simulink model "fault_tolerant_controller_2014"  (R2014a)
settings: Solver=ode45  SolverMode=SingleTasking  StartTime=0.0  StopTime=150  RelTol=1e-3
values from neighbouring files (symbols this model uses):
  g = 9.8    [model.mat]
  Kd = 1e-06    [model.mat]
  Kt = 1    [model.mat]
  U0 = 120    [model.mat]
  X0 = 0    [model.mat]
  Y0 = 5000    [model.mat]
undefined symbols (not defined in the file or in its folder): magnitude
libraries: simulink x53, aerolibatmos2 x12, aerolibconvert2 x4
(part 2 of 2)

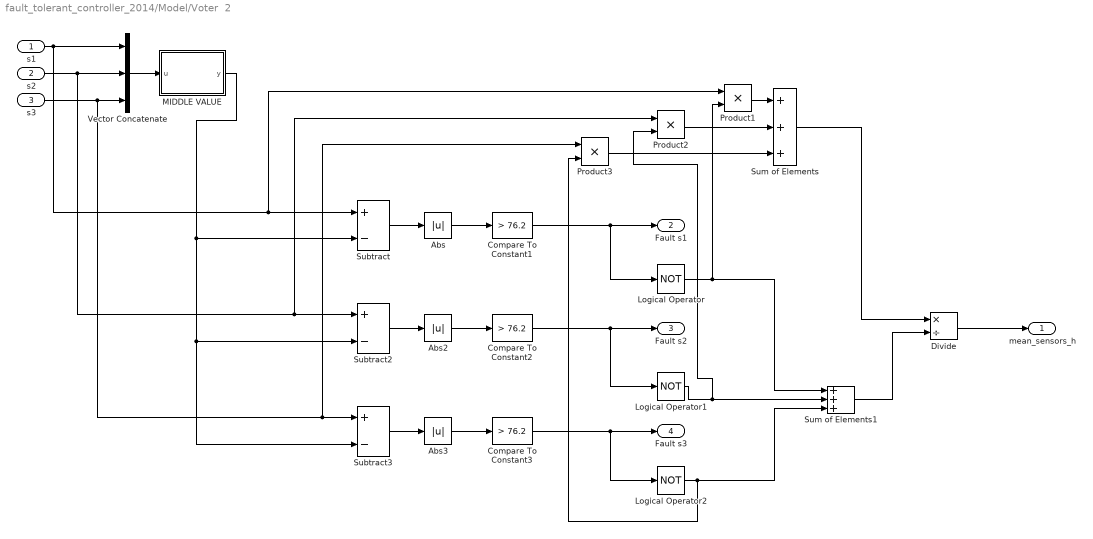
== system fault_tolerant_controller_2014/Model/Voter  2 ==
  s1 : Inport
  s2 : Inport  Port=2
  s3 : Inport  Port=3
  Abs : Abs
  Abs2 : Abs
  Abs3 : Abs
  Compare To Constant1 : simulink/Logic and Bit Operations/Compare To Constant  relop=>  const=76.2  OutDataTypeStr=boolean
  Compare To Constant2 : simulink/Logic and Bit Operations/Compare To Constant  relop=>  const=76.2  OutDataTypeStr=boolean
  Compare To Constant3 : simulink/Logic and Bit Operations/Compare To Constant  relop=>  const=76.2  OutDataTypeStr=boolean
  Divide : Product  Inputs=*/
  Logical Operator : Logic  Operator=NOT  AllPortsSameDT=off  OutDataTypeStr=boolean
  Logical Operator1 : Logic  Operator=NOT  AllPortsSameDT=off  OutDataTypeStr=boolean
  Logical Operator2 : Logic  Operator=NOT  AllPortsSameDT=off  OutDataTypeStr=boolean
  "MIDDLE VALUE " : MATLAB Function  TreatAsAtomicUnit=on
      settings: PermitHierarchicalResolution=ParametersOnly
  Product1 : Product
  Product2 : Product
  Product3 : Product
  Subtract : Sum  Inputs=+-
  Subtract2 : Sum  Inputs=+-
  Subtract3 : Sum  Inputs=+-
  Sum of Elements : Sum  Inputs=+++
  Sum of Elements1 : Sum  Inputs=+++
  Vector Concatenate : Concatenate  NumInputs=3
  " mean_sensors_h" : Outport
  "Fault s1  " : Outport  Port=2
  "Fault s2  " : Outport  Port=3
  "Fault s3  " : Outport  Port=4
  wires:
  Vector Concatenate/1 -> "MIDDLE VALUE "/1(u)
  Subtract3/1 -> Abs3/1
  Subtract/1 -> Abs/1
  s3/1 -> Product3/1, Subtract3/1, Vector Concatenate/3
  Subtract2/1 -> Abs2/1
  "MIDDLE VALUE "/1(y) -> Subtract/2, Subtract3/2, Subtract2/2
  Sum of Elements/1 -> Divide/1
  Sum of Elements1/1 -> Divide/2
  Divide/1 -> " mean_sensors_h"/1
  Abs/1 -> Compare To Constant1/1
  Compare To Constant1/1 -> Logical Operator/1, "Fault s1  "/1
  Compare To Constant2/1 -> Logical Operator1/1, "Fault s2  "/1
  Abs2/1 -> Compare To Constant2/1
  Abs3/1 -> Compare To Constant3/1
  Compare To Constant3/1 -> Logical Operator2/1, "Fault s3  "/1
  Logical Operator/1 -> Product1/2, Sum of Elements1/1
  Logical Operator1/1 -> Sum of Elements1/2, Product2/2
  Logical Operator2/1 -> Sum of Elements1/3, Product3/2
  s1/1 -> Product1/1, Subtract/1, Vector Concatenate/1
  s2/1 -> Product2/1, Subtract2/1, Vector Concatenate/2
  Product2/1 -> Sum of Elements/2
  Product3/1 -> Sum of Elements/3
  Product1/1 -> Sum of Elements/1

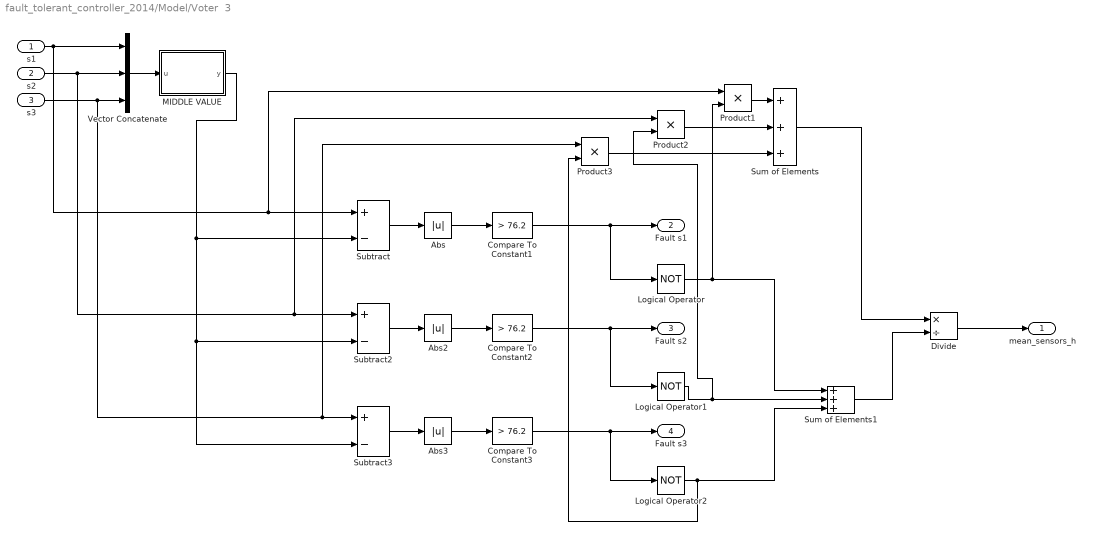
== system fault_tolerant_controller_2014/Model/Voter  3 ==
  s1 : Inport
  s2 : Inport  Port=2
  s3 : Inport  Port=3
  Abs : Abs
  Abs2 : Abs
  Abs3 : Abs
  Compare To Constant1 : simulink/Logic and Bit Operations/Compare To Constant  relop=>  const=76.2  OutDataTypeStr=boolean
  Compare To Constant2 : simulink/Logic and Bit Operations/Compare To Constant  relop=>  const=76.2  OutDataTypeStr=boolean
  Compare To Constant3 : simulink/Logic and Bit Operations/Compare To Constant  relop=>  const=76.2  OutDataTypeStr=boolean
  Divide : Product  Inputs=*/
  Logical Operator : Logic  Operator=NOT  AllPortsSameDT=off  OutDataTypeStr=boolean
  Logical Operator1 : Logic  Operator=NOT  AllPortsSameDT=off  OutDataTypeStr=boolean
  Logical Operator2 : Logic  Operator=NOT  AllPortsSameDT=off  OutDataTypeStr=boolean
  "MIDDLE VALUE " : MATLAB Function  TreatAsAtomicUnit=on
      settings: PermitHierarchicalResolution=ParametersOnly
  Product1 : Product
  Product2 : Product
  Product3 : Product
  Subtract : Sum  Inputs=+-
  Subtract2 : Sum  Inputs=+-
  Subtract3 : Sum  Inputs=+-
  Sum of Elements : Sum  Inputs=+++
  Sum of Elements1 : Sum  Inputs=+++
  Vector Concatenate : Concatenate  NumInputs=3
  " mean_sensors_h" : Outport
  "Fault s1  " : Outport  Port=2
  "Fault s2  " : Outport  Port=3
  "Fault s3  " : Outport  Port=4
  wires:
  Vector Concatenate/1 -> "MIDDLE VALUE "/1(u)
  Subtract3/1 -> Abs3/1
  Subtract/1 -> Abs/1
  s3/1 -> Product3/1, Subtract3/1, Vector Concatenate/3
  Subtract2/1 -> Abs2/1
  "MIDDLE VALUE "/1(y) -> Subtract/2, Subtract3/2, Subtract2/2
  Sum of Elements/1 -> Divide/1
  Sum of Elements1/1 -> Divide/2
  Divide/1 -> " mean_sensors_h"/1
  Abs/1 -> Compare To Constant1/1
  Compare To Constant1/1 -> Logical Operator/1, "Fault s1  "/1
  Compare To Constant2/1 -> Logical Operator1/1, "Fault s2  "/1
  Abs2/1 -> Compare To Constant2/1
  Abs3/1 -> Compare To Constant3/1
  Compare To Constant3/1 -> Logical Operator2/1, "Fault s3  "/1
  Logical Operator/1 -> Product1/2, Sum of Elements1/1
  Logical Operator1/1 -> Sum of Elements1/2, Product2/2
  Logical Operator2/1 -> Sum of Elements1/3, Product3/2
  s1/1 -> Product1/1, Subtract/1, Vector Concatenate/1
  s2/1 -> Product2/1, Subtract2/1, Vector Concatenate/2
  Product2/1 -> Sum of Elements/2
  Product3/1 -> Sum of Elements/3
  Product1/1 -> Sum of Elements/1

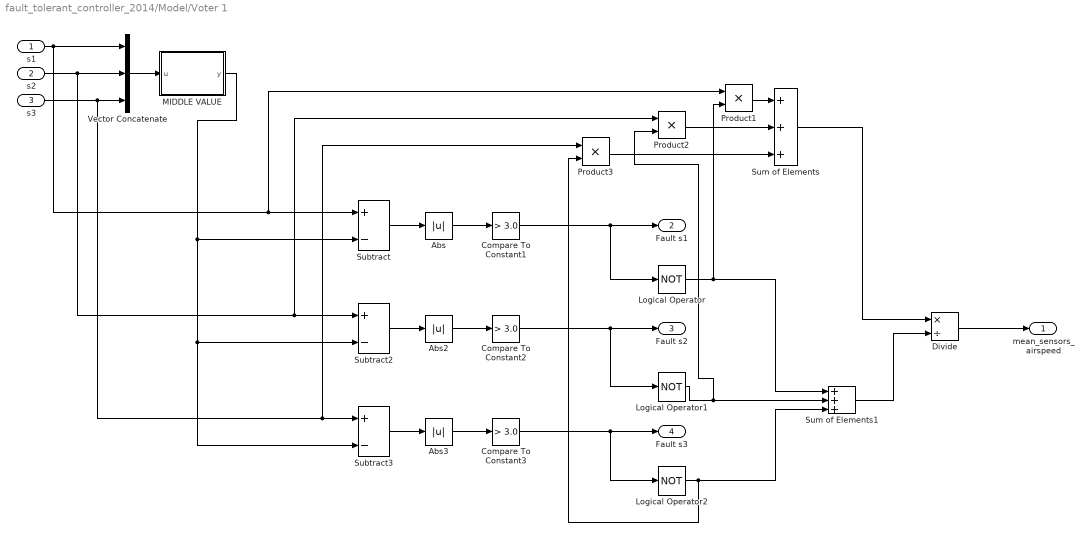
== system fault_tolerant_controller_2014/Model/Voter 1 ==
  s1 : Inport
  s2 : Inport  Port=2
  s3 : Inport  Port=3
  Abs : Abs
  Abs2 : Abs
  Abs3 : Abs
  Compare To Constant1 : simulink/Logic and Bit Operations/Compare To Constant  relop=>  const=3.0  OutDataTypeStr=boolean
  Compare To Constant2 : simulink/Logic and Bit Operations/Compare To Constant  relop=>  const=3.0  OutDataTypeStr=boolean
  Compare To Constant3 : simulink/Logic and Bit Operations/Compare To Constant  relop=>  const=3.0  OutDataTypeStr=boolean
  Divide : Product  Inputs=*/
  Logical Operator : Logic  Operator=NOT  AllPortsSameDT=off  OutDataTypeStr=boolean
  Logical Operator1 : Logic  Operator=NOT  AllPortsSameDT=off  OutDataTypeStr=boolean
  Logical Operator2 : Logic  Operator=NOT  AllPortsSameDT=off  OutDataTypeStr=boolean
  "MIDDLE VALUE " : MATLAB Function  TreatAsAtomicUnit=on
      settings: PermitHierarchicalResolution=ParametersOnly
  Product1 : Product
  Product2 : Product
  Product3 : Product
  Subtract : Sum  Inputs=+-
  Subtract2 : Sum  Inputs=+-
  Subtract3 : Sum  Inputs=+-
  Sum of Elements : Sum  Inputs=+++
  Sum of Elements1 : Sum  Inputs=+++
  Vector Concatenate : Concatenate  NumInputs=3
  " mean_sensors_airspeed" : Outport
  "Fault s1  " : Outport  Port=2
  "Fault s2  " : Outport  Port=3
  "Fault s3  " : Outport  Port=4
  wires:
  Vector Concatenate/1 -> "MIDDLE VALUE "/1(u)
  Subtract3/1 -> Abs3/1
  Subtract/1 -> Abs/1
  s3/1 -> Product3/1, Subtract3/1, Vector Concatenate/3
  Subtract2/1 -> Abs2/1
  "MIDDLE VALUE "/1(y) -> Subtract/2, Subtract3/2, Subtract2/2
  Sum of Elements/1 -> Divide/1
  Sum of Elements1/1 -> Divide/2
  Divide/1 -> " mean_sensors_airspeed"/1
  Abs/1 -> Compare To Constant1/1
  Compare To Constant1/1 -> Logical Operator/1, "Fault s1  "/1
  Compare To Constant2/1 -> Logical Operator1/1, "Fault s2  "/1
  Abs2/1 -> Compare To Constant2/1
  Abs3/1 -> Compare To Constant3/1
  Compare To Constant3/1 -> Logical Operator2/1, "Fault s3  "/1
  Logical Operator/1 -> Product1/2, Sum of Elements1/1
  Logical Operator1/1 -> Sum of Elements1/2, Product2/2
  Logical Operator2/1 -> Sum of Elements1/3, Product3/2
  s1/1 -> Product1/1, Subtract/1, Vector Concatenate/1
  s2/1 -> Product2/1, Subtract2/1, Vector Concatenate/2
  Product2/1 -> Sum of Elements/2
  Product3/1 -> Sum of Elements/3
  Product1/1 -> Sum of Elements/1

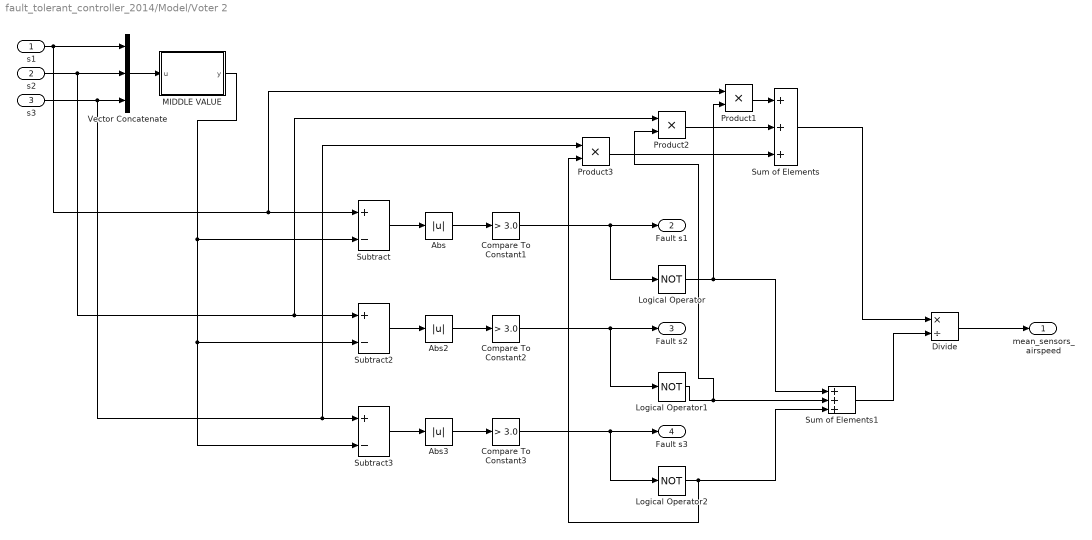
== system fault_tolerant_controller_2014/Model/Voter 2 ==
  s1 : Inport
  s2 : Inport  Port=2
  s3 : Inport  Port=3
  Abs : Abs
  Abs2 : Abs
  Abs3 : Abs
  Compare To Constant1 : simulink/Logic and Bit Operations/Compare To Constant  relop=>  const=3.0  OutDataTypeStr=boolean
  Compare To Constant2 : simulink/Logic and Bit Operations/Compare To Constant  relop=>  const=3.0  OutDataTypeStr=boolean
  Compare To Constant3 : simulink/Logic and Bit Operations/Compare To Constant  relop=>  const=3.0  OutDataTypeStr=boolean
  Divide : Product  Inputs=*/
  Logical Operator : Logic  Operator=NOT  AllPortsSameDT=off  OutDataTypeStr=boolean
  Logical Operator1 : Logic  Operator=NOT  AllPortsSameDT=off  OutDataTypeStr=boolean
  Logical Operator2 : Logic  Operator=NOT  AllPortsSameDT=off  OutDataTypeStr=boolean
  "MIDDLE VALUE " : MATLAB Function  TreatAsAtomicUnit=on
      settings: PermitHierarchicalResolution=ParametersOnly
  Product1 : Product
  Product2 : Product
  Product3 : Product
  Subtract : Sum  Inputs=+-
  Subtract2 : Sum  Inputs=+-
  Subtract3 : Sum  Inputs=+-
  Sum of Elements : Sum  Inputs=+++
  Sum of Elements1 : Sum  Inputs=+++
  Vector Concatenate : Concatenate  NumInputs=3
  " mean_sensors_airspeed" : Outport
  "Fault s1  " : Outport  Port=2
  "Fault s2  " : Outport  Port=3
  "Fault s3  " : Outport  Port=4
  wires:
  Vector Concatenate/1 -> "MIDDLE VALUE "/1(u)
  Subtract3/1 -> Abs3/1
  Subtract/1 -> Abs/1
  s3/1 -> Product3/1, Subtract3/1, Vector Concatenate/3
  Subtract2/1 -> Abs2/1
  "MIDDLE VALUE "/1(y) -> Subtract/2, Subtract3/2, Subtract2/2
  Sum of Elements/1 -> Divide/1
  Sum of Elements1/1 -> Divide/2
  Divide/1 -> " mean_sensors_airspeed"/1
  Abs/1 -> Compare To Constant1/1
  Compare To Constant1/1 -> Logical Operator/1, "Fault s1  "/1
  Compare To Constant2/1 -> Logical Operator1/1, "Fault s2  "/1
  Abs2/1 -> Compare To Constant2/1
  Abs3/1 -> Compare To Constant3/1
  Compare To Constant3/1 -> Logical Operator2/1, "Fault s3  "/1
  Logical Operator/1 -> Product1/2, Sum of Elements1/1
  Logical Operator1/1 -> Sum of Elements1/2, Product2/2
  Logical Operator2/1 -> Sum of Elements1/3, Product3/2
  s1/1 -> Product1/1, Subtract/1, Vector Concatenate/1
  s2/1 -> Product2/1, Subtract2/1, Vector Concatenate/2
  Product2/1 -> Sum of Elements/2
  Product3/1 -> Sum of Elements/3
  Product1/1 -> Sum of Elements/1

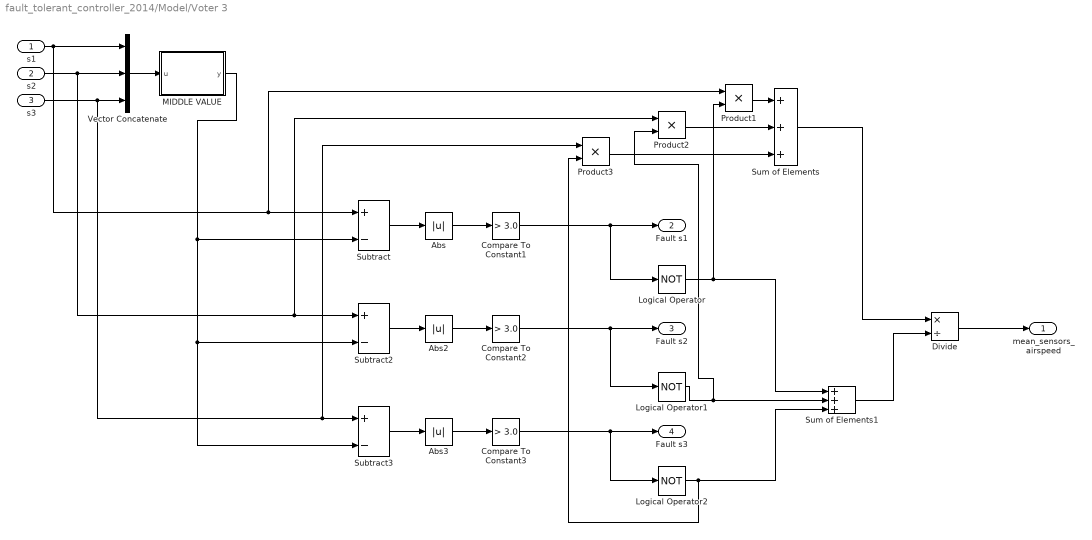
== system fault_tolerant_controller_2014/Model/Voter 3   ==
  s1 : Inport
  s2 : Inport  Port=2
  s3 : Inport  Port=3
  Abs : Abs
  Abs2 : Abs
  Abs3 : Abs
  Compare To Constant1 : simulink/Logic and Bit Operations/Compare To Constant  relop=>  const=3.0  OutDataTypeStr=boolean
  Compare To Constant2 : simulink/Logic and Bit Operations/Compare To Constant  relop=>  const=3.0  OutDataTypeStr=boolean
  Compare To Constant3 : simulink/Logic and Bit Operations/Compare To Constant  relop=>  const=3.0  OutDataTypeStr=boolean
  Divide : Product  Inputs=*/
  Logical Operator : Logic  Operator=NOT  AllPortsSameDT=off  OutDataTypeStr=boolean
  Logical Operator1 : Logic  Operator=NOT  AllPortsSameDT=off  OutDataTypeStr=boolean
  Logical Operator2 : Logic  Operator=NOT  AllPortsSameDT=off  OutDataTypeStr=boolean
  "MIDDLE VALUE " : MATLAB Function  TreatAsAtomicUnit=on
      settings: PermitHierarchicalResolution=ParametersOnly
  Product1 : Product
  Product2 : Product
  Product3 : Product
  Subtract : Sum  Inputs=+-
  Subtract2 : Sum  Inputs=+-
  Subtract3 : Sum  Inputs=+-
  Sum of Elements : Sum  Inputs=+++
  Sum of Elements1 : Sum  Inputs=+++
  Vector Concatenate : Concatenate  NumInputs=3
  " mean_sensors_airspeed" : Outport
  "Fault s1  " : Outport  Port=2
  "Fault s2  " : Outport  Port=3
  "Fault s3  " : Outport  Port=4
  wires:
  Vector Concatenate/1 -> "MIDDLE VALUE "/1(u)
  Subtract3/1 -> Abs3/1
  Subtract/1 -> Abs/1
  s3/1 -> Product3/1, Subtract3/1, Vector Concatenate/3
  Subtract2/1 -> Abs2/1
  "MIDDLE VALUE "/1(y) -> Subtract/2, Subtract3/2, Subtract2/2
  Sum of Elements/1 -> Divide/1
  Sum of Elements1/1 -> Divide/2
  Divide/1 -> " mean_sensors_airspeed"/1
  Abs/1 -> Compare To Constant1/1
  Compare To Constant1/1 -> Logical Operator/1, "Fault s1  "/1
  Compare To Constant2/1 -> Logical Operator1/1, "Fault s2  "/1
  Abs2/1 -> Compare To Constant2/1
  Abs3/1 -> Compare To Constant3/1
  Compare To Constant3/1 -> Logical Operator2/1, "Fault s3  "/1
  Logical Operator/1 -> Product1/2, Sum of Elements1/1
  Logical Operator1/1 -> Sum of Elements1/2, Product2/2
  Logical Operator2/1 -> Sum of Elements1/3, Product3/2
  s1/1 -> Product1/1, Subtract/1, Vector Concatenate/1
  s2/1 -> Product2/1, Subtract2/1, Vector Concatenate/2
  Product2/1 -> Sum of Elements/2
  Product3/1 -> Sum of Elements/3
  Product1/1 -> Sum of Elements/1

== system fault_tolerant_controller_2014/Model/plant  ==
  dt : Inport
  "gamma " : Inport  Port=2
  Gain : Gain  Gain=g
  Integrator : Integrator  InitialCondition=U0
  Integrator1 : Integrator  InitialCondition=X0
  Integrator2 : Integrator  InitialCondition=Y0
  Kd : Gain  Gain=Kd
  Kt : Gain  Gain=Kt
  "MIDDLE VALUE " : MATLAB Function  TreatAsAtomicUnit=on
      settings: PermitHierarchicalResolution=ParametersOnly
  MIDDLE VALUE 1 : MATLAB Function  TreatAsAtomicUnit=on
      settings: PermitHierarchicalResolution=ParametersOnly
  Math Function : Math  Operator=magnitude^2  SaturateOnIntegerOverflow=on
  Product : Product
  Product1 : Product
  Rate Limiter : RateLimiter  RisingSlewLimit=pi/180  FallingSlewLimit=-pi/180  SampleTimeMode=inherited
  Saturation : Saturate  UpperLimit=15  LowerLimit=0
  Scope : Scope  NumInputPorts=3
      settings: TimeRange=auto  MaxDataPoints=5000  SaveToWorkspace=off  YMin=-0.08421~-0.06411~-0.00654  YMax=0.7579~0.577~0.0589  SampleTime=-1
  Sum : Sum  Inputs=-+-
  Trigonometric Function : Trigonometry
  Trigonometric Function1 : Trigonometry  Operator=cos
  Airspeed : Outport
  x : Outport  Port=2
  y : Outport  Port=3
  wires:
  Integrator/1 -> Product/1, Math Function/1, Airspeed/1, Product1/1
  Product/1 -> Integrator2/1
  Integrator1/1 -> x/1
  Trigonometric Function1/1 -> Product1/2
  Product1/1 -> Integrator1/1
  Trigonometric Function/1 -> Gain/1, Product/2
  Integrator2/1 -> y/1
  Sum/1 -> Scope/1, Integrator/1
  Kt/1 -> Saturation/1
  Kd/1 -> Sum/1
  Math Function/1 -> Kd/1
  Gain/1 -> Sum/3
  Rate Limiter/1 -> Scope/3, Trigonometric Function1/1, Trigonometric Function/1
  Saturation/1 -> Scope/2, Sum/2
  dt/1 -> "MIDDLE VALUE "/1(u)
  "MIDDLE VALUE "/1(y) -> Kt/1
  MIDDLE VALUE 1/1(y) -> Rate Limiter/1
  "gamma "/1 -> MIDDLE VALUE 1/1(u)

== matlab function fault_tolerant_controller_2014/Model/Voter 3  /MIDDLE VALUE  ==
  data: u input; y output
function y = fcn(u)

y = median(u);

== matlab function fault_tolerant_controller_2014/Model/Voter  1/MIDDLE VALUE  ==
  data: u input; y output
function y = fcn(u)

y = median(u);

== matlab function fault_tolerant_controller_2014/Model/Voter 1/MIDDLE VALUE  ==
  data: u input; y output
function y = fcn(u)

y = median(u);

== matlab function fault_tolerant_controller_2014/Model/Voter  2/MIDDLE VALUE  ==
  data: u input; y output
function y = fcn(u)

y = median(u);

== matlab function fault_tolerant_controller_2014/Model/Voter  3/MIDDLE VALUE  ==
  data: u input; y output
function y = fcn(u)

y = median(u);

== matlab function fault_tolerant_controller_2014/Model/Voter 2/MIDDLE VALUE  ==
  data: u input; y output
function y = fcn(u)

y = median(u);

== matlab function fault_tolerant_controller_2014/Model/plant /MIDDLE VALUE  ==
  data: u input; y output
function y = fcn(u)

y = median(u);

== matlab function fault_tolerant_controller_2014/Model/plant /MIDDLE VALUE 1 ==
  data: u input; y output
function y = fcn(u)

y = median(u);
